simulink model "V3"  (R2024b)
settings: Solver=ode1  StartTime=0.0  StopTime=inf  FixedStep=0.1  RelTol=1e-3  EnableMultiTasking=on
PostLoadFcn:
  | qlabs_setup
model workspace (MAT data in the model file):
  Sig : Simulink.Signal (value not decoded)
  downCamStepSize : Simulink.Parameter (value not decoded)
  lidarStepSize : Simulink.Parameter (value not decoded)
  mainStepSize : Simulink.Parameter (value not decoded)
  mode : Simulink.Parameter (value not decoded)
  realSenseStepSize : Simulink.Parameter (value not decoded)
values from neighbouring files (symbols this model uses):
  map = zeros(mapHeight*pointPerMeter, mapWidth*pointPerMeter)    [map_creator.m]    (also in map_creator_real.m)
  obstacles = [obstacles; coordinateX, coordinateY, rayon;]    [init.m]    (also in init1.m; init_V2.m; init_V3.m; map_creator.m = [)
  pointPerMeter = 50    [map_creator.m]    (also in map_creator_real.m)
  waypoints = [ ... (first row only)    [init.m]    (also in init1.m; init_V2.m; init_V3.m)
  x = input("Veuillez entrer la position x: ")    [map_creator_real.m]
symbols that are objects in the model workspace (value not decoded): downCamStepSize, lidarStepSize, mainStepSize, realSenseStepSize
undefined symbols (not defined in the file or in its folder): DiscIntNeverNeededParam, gcbh, JPEG, Point, qc_get_step_size, Video3D, video_display_show
libraries: quarc_library x30, mpclib x1, simulink_extras x1
(part 2 of 2)

== matlab function V3/LiDAR analysis1/Grid matching ==
  data: map input; x_rob input; y_rob input; scan_ranges input; scan_angles input; theta_opt output double; theta_prec input; pointPerMeter input
function theta_opt = estimate_heading_optimized(map, x_rob, y_rob, scan_ranges, scan_angles, theta_prec, pointPerMeter)
    % map         : Matrice 2D (occupancy grid) avec des valeurs entre 0 et 1
    % x_rob, y_rob: Coordonnées actuelles du robot en mètres 
    % scan_ranges : Vecteur colonne des distances LiDAR (en mètres)
    % scan_angles : Vecteur colonne des angles du LiDAR correspondants (en radians)
    % theta_prec  : Dernier angle connu ou estimé du robot (en radians)
    
    % --- Paramètres fixes ---
    cell_size = 1/pointPerMeter; % 2 cm par case
    [rows, cols] = size(map);
    
    % Centre de la matrice (correspondant à x=0, y=0)
    cx = floor(cols / 2) + 1;
    cy = floor(rows / 2) + 1; 
    
    % --- Espace de recherche restreint ---
    % On cherche de -30° à +30° autour de theta_prec avec un pas de 1°
    % Cela donne exactement 61 valeurs à tester.
    num_steps = 61;
    angle_step = pi / 180; % 1 degré en radians
    start_angle = theta_prec - (30 * angle_step);
    
    max_score = -1;
    theta_opt = theta_prec; % Si le scan est vide, on renvoie l'ancien angle
    
    % --- Boucle de Scan Matching ---
    for i = 1:num_steps
        % Calcul de l'angle testé à la volée (évite les vecteurs de taille variable)
        theta = start_angle + (i - 1) * angle_step;
        current_score = 0;
        
        % On parcourt chaque point du scan LiDAR
        for j = 1:length(scan_ranges)
            range = scan_ranges(j);
            
            % Filtrage des valeurs invalides du capteur (0 ou trop loin)
            if range > 0 && range < 100 
                angle = scan_angles(j);
                
                % 1. Coordonnées globales en mètres
                hit_x_m = x_rob + range * cos(angle + theta);
                hit_y_m = y_rob + range * sin(angle + theta);
                
                % 2. Conversion en indices de la matrice (Y inversé)
                idx_x = cx + round(hit_x_m / cell_size);
                idx_y = cy - round(hit_y_m / cell_size); 
                
                % 3. Vérification des limites pour éviter un crash
                if idx_x >= 1 && idx_x <= cols && idx_y >= 1 && idx_y <= rows
                    % Ajout de la valeur de la case au score de cet angle
                    current_score = current_score + map(idx_y, idx_x);
                end
            end
        end
        
        % 4. Sauvegarde de l'angle si c'est le meilleur score jusqu'à présent
        if current_score > max_score
            max_score = current_score;
            theta_opt = theta;
        end
    end
end

== matlab function V3/LiDAR analysis1/Lidar & Localization/MATLAB Function ==
  data: lidar_position input; ranges input; ranges_c output; angles input; angles_c output
function [ranges_c,angles_c] = correct_lidar(lidar_position, ranges,angles)

x = ranges.*cos(angles) + lidar_position(1);
y = ranges.*sin(angles) + lidar_position(2);

ranges_c = sqrt(x.^2 + y.^2);
angles_c = atan2(y, x);

end

== matlab function V3/MATLAB Function1 ==
  data: t input; X_ref output size=[3, 25]; obstacles input; waypoints input; is_final_approach output
function [X_ref, is_final_approach] = Traj_bezier_horizon(t, obstacles, waypoints)
    % Entrées : 
    %   t          : Temps de simulation actuel (secondes)
    %   obstacles  : Matrice des obstacles [x, y, rayon]
    %   waypoints  : Matrice des points de passage [x, y, theta]
    % Sorties : 
    %   X_ref            : Matrice [3 x Np] contenant les références futures [x; y; theta]
    %   kappa_actuel     : Scalaire de la courbure locale à l'instant t
    %   is_final_approach: Flag (0 ou 1) indiquant l'approche finale

    coder.extrinsic('plot', 'fill', 'quiver', 'figure', 'unwrap', 'warning');

    Ts = 0.1;   % Pas de temps 
    Np = 25;  

    X_ref             = zeros(3, Np);
    kappa_actuel      = 0;
    is_final_approach = 0;

    % Mémoire persistante avec types explicites pour le Coder
    persistent time_ref x_ref y_ref theta_ref kappa_ref initialized

    if isempty(initialized)
        initialized = int32(0);
        v_max = 0.5;
        omega_max = 2.0; 

        obstacles_rect   = [];
        n_points_per_seg = 1000;
        marge_securite   = 0.6;

        % typée double(0x1) pour que le Coder Simulink puisse inférer le type correctement
        x_total     = zeros(0, 1);
        y_total     = zeros(0, 1);
        theta_total = zeros(0, 1);
        kappa_total = zeros(0, 1);
        time_total  = zeros(0, 1);
        cumul_time  = 0;

        for seg = 1:(size(waypoints, 1) - 1)

            x_start = waypoints(seg,   1);  y_start = waypoints(seg,   2);  theta_start = waypoints(seg,   3);
            x_goal  = waypoints(seg+1, 1);  y_goal  = waypoints(seg+1, 2);  theta_goal  = waypoints(seg+1, 3);

            distance = sqrt((x_goal - x_start)^2 + (y_goal - y_start)^2);
            if distance < 1e-3
                warning('Traj_bezier_horizon: segment %d ignoré (distance < 1e-3).', seg);
                continue;
            end

            longueur_tangente = distance / 3;

            P0 = [x_start, y_start];
            P1 = P0 + longueur_tangente * [cos(theta_start), sin(theta_start)];
            P2 = [x_goal, y_goal] - longueur_tangente * [cos(theta_goal), sin(theta_goal)];
            P3 = [x_goal, y_goal];

            % Répulsion des points de contrôle vis-à-vis des obstacles circulaires
            for i = 1:size(obstacles, 1)
                obs_c = obstacles(i, 1:2);
                r_obs = obstacles(i, 3);

                if norm(P1 - obs_c) < r_obs + marge_securite + 0.5
                    dir = (P1 - obs_c) / norm(P1 - obs_c);
                    P1  = obs_c + dir * (r_obs + marge_securite + 0.2);
                end
                if norm(P2 - obs_c) < r_obs + marge_securite + 0.5
                    dir = (P2 - obs_c) / norm(P2 - obs_c);
                    P2  = obs_c + dir * (r_obs + marge_securite + 0.8);
                end
            end

            % Répulsion vis-à-vis des obstacles rectangulaires
            for i = 1:size(obstacles_rect, 1)
                xc  = obstacles_rect(i, 1);  yc  = obstacles_rect(i, 2);
                W   = obstacles_rect(i, 3);  H   = obstacles_rect(i, 4);
                ang = obstacles_rect(i, 5);
                R_mat       = [cos(ang), -sin(ang); sin(ang), cos(ang)];
                corners_loc = [-W/2, -H/2; W/2, -H/2; W/2, H/2; -W/2, H/2];
                corners_glob = (R_mat * corners_loc')' + [xc, yc];
                r_coin = 0.3;

                for j = 1:4
                    coin = corners_glob(j, :);
                    if norm(P1 - coin) < r_coin + marge_securite + 0.5
                        dir = (P1 - coin) / norm(P1 - coin);
                        P1  = coin + dir * (r_coin + marge_securite + 0.8);
                    end
                    if norm(P2 - coin) < r_coin + marge_securite + 0.5
                        dir = (P2 - coin) / norm(P2 - coin);
                        P2  = coin + dir * (r_coin + marge_securite + 0.8);
                    end
                end
            end

            % Génération de la courbe de Bézier cubique
            tt    = linspace(0, 1, n_points_per_seg)';
            x_seg = (1-tt).^3*P0(1) + 3*(1-tt).^2.*tt*P1(1) + 3*(1-tt).*tt.^2*P2(1) + tt.^3*P3(1);
            y_seg = (1-tt).^3*P0(2) + 3*(1-tt).^2.*tt*P1(2) + 3*(1-tt).*tt.^2*P2(2) + tt.^3*P3(2);

            dx  = gradient(x_seg);
            dy  = gradient(y_seg);
            ddx = gradient(dx);
            ddy = gradient(dy);

            theta_seg = atan2(dy, dx);
            kappa     = (dx.*ddy - dy.*ddx) ./ ((dx.^2 + dy.^2).^(3/2) + 1e-6);
            kappa(isnan(kappa)) = 0;

            % Profil de vitesse adaptatif (ralentissement dans les virages)
            v_seg = v_max * ones(size(kappa));
            for k = 1:length(kappa)
                if abs(kappa(k)) > 0.01
                    v_lim    = sqrt(3.0 / abs(kappa(k)));
                    v_seg(k) = min(v_seg(k), v_lim);
                end
            end
            v_seg = min(v_seg, v_max);

            % Conversion paramètre [0,1] → temps réel
            ds       = [0; sqrt(diff(x_seg).^2 + diff(y_seg).^2)];
            dt_seg   = ds ./ max(v_seg, 0.01);
            time_seg = cumsum(dt_seg) + cumul_time;

            if seg == 1
                x_total     = [x_total;     x_seg];     
                y_total     = [y_total;     y_seg];     
                theta_total = [theta_total; theta_seg]; 
                kappa_total = [kappa_total; kappa];     
                time_total  = [time_total;  time_seg]; 
            else
                x_total     = [x_total;     x_seg(2:end)];     
                y_total     = [y_total;     y_seg(2:end)];     
                theta_total = [theta_total; theta_seg(2:end)];
                kappa_total = [kappa_total; kappa(2:end)];     
                time_total  = [time_total;  time_seg(2:end)];  
            end

            cumul_time = time_total(end);
        end
        
        % theta_total = unwrap(theta_total);

        % Stockage persistant
        time_ref  = time_total;
        x_ref     = x_total;
        y_ref     = y_total;
        theta_ref = theta_total;
        kappa_ref = kappa_total;

        % Tracé debug
        figure('Name', 'Trajectoire Bézier MPC', 'Position', [970 100 900 700]);
        hold on; grid on; axis equal;
        for i = 1:size(obstacles, 1)
            circle_x = obstacles(i,1) + obstacles(i,3) * cos(0:0.01:2*pi);
            circle_y = obstacles(i,2) + obstacles(i,3) * sin(0:0.01:2*pi);
            fill(circle_x, circle_y, [1 0.7 0.7], 'EdgeColor', 'r', 'LineWidth', 2);
        end
        plot(x_ref, y_ref, 'b-', 'LineWidth', 3);

        initialized = int32(1);

        % Au tout premier appel on retourne immédiatement les valeurs
        % par défaut déjà initialisées en tête (t=0 → pas encore de
        % trajectoire à interpoler de façon significative).

        return;
    end

    % ==========================================================
    % PHASE 2 : CALCUL DE LA MATRICE DE RÉFÉRENCE SUR L'HORIZON
    % ==========================================================

    % =========================================================
    % ARRÊT : on calcule la distance à l'arrivée en temps réel
    % à partir de la position estimée du robot (x_init passé en
    % entrée depuis le bloc MPC) mais ici on n'a pas x_init.
    % On utilise donc une double condition :
    %   - temporelle  : t > time_ref(end) - marge
    %   - ET spatiale : sera vérifiée côté MPC avec x_init réel
    % On réduit la marge temporelle à 0.5 s (au lieu de 2 s) pour
    % ne déclencher "final" qu'au dernier moment.
    % =========================================================
    dist_to_goal_ref = sqrt((interp1(time_ref, x_ref, min(t, time_ref(end)), 'linear') - x_ref(end))^2 + ...
                            (interp1(time_ref, y_ref, min(t, time_ref(end)), 'linear') - y_ref(end))^2);

    if t > (time_ref(end) - 0.5) || dist_to_goal_ref < 0.3
        is_final_approach = 1;
    else
        is_final_approach = 0;
    end

    if t > time_ref(end)
        % Fin de trajectoire : on reste sur la dernière pose
        X_ref(1, :) = x_ref(end);
        X_ref(2, :) = y_ref(end);
        X_ref(3, :) = theta_ref(end);
        kappa_actuel = 0;
    else
        t_horizon        = t + (0:Np-1) * Ts;
        t_horizon_capped = min(t_horizon, time_ref(end));

        xr_vec     = interp1(time_ref, x_ref,     t_horizon_capped, 'linear');
        yr_vec     = interp1(time_ref, y_ref,     t_horizon_capped, 'linear');
        thetar_vec = interp1(time_ref, theta_ref, t_horizon_capped, 'linear');

        X_ref(1, :) = xr_vec;
        X_ref(2, :) = yr_vec;
        X_ref(3, :) = thetar_vec;

        kappa_actuel = interp1(time_ref, kappa_ref, t, 'spline');
    end
end

== matlab function V3/V1 ==
  data: obstacles input; X_ref input; u_prev input; kappa input; x_init input; u_opt output
function u_opt = Matisse_MPC_Quanser(obstacles, X_ref, u_prev, kappa, x_init)
    % Déclaration pour autoriser les fonctions d'optimisation dans Simulink
    coder.extrinsic('fmincon', 'optimoptions');
    
    % --- Paramètres constants ---
    Np = 12; 
    Ts = 0.1;
    v_max = 0.5;
    w_max = 2.0;
    
    % --- ADAPTATION DYNAMIQUE MATISSE ---
    % 1. Adaptation Géométrique (Courbure)
    Q = diag([10, 10, 5 * (1 + abs(kappa))]); 
    
    % 2. Adaptation Réactive (Obstacles)
    % On cherche la distance à l'obstacle le plus proche
    d_min = 10.0; % Valeur grande par défaut
    if ~isempty(obstacles)
        for j = 1:size(obstacles, 1)
            dist = norm(x_init(1:2) - obstacles(j, 1:2)) - obstacles(j, 3);
            if dist < d_min
                d_min = dist;
            end
        end
    end
    
    % Si l'obstacle est proche, on réduit R pour autoriser une forte accélération
    R_nom = diag([0.1, 0.05]);
    R = R_nom * tanh(max(d_min, 0.1)); 
    
    S = diag([0.5, 0.5]); % Poids sur le lissage (Delta U)
    P = Q * 10;           % Coût terminal pour la stabilité

    % --- BORNES (Limites des moteurs) ---
    % lb et ub doivent être de taille [2*Np, 1]
    lb = repmat([-v_max; -w_max], Np, 1);
    ub = repmat([v_max; w_max], Np, 1);

    % --- OPTIMISATION ---
    % Initialisation avec la commande précédente (Warm Start)
    u0 = repmat(u_prev, Np, 1);
    
    % Options du solveur
    options = optimoptions('fmincon', 'Algorithm', 'sqp', 'Display', 'off');
    
    % Valeur par défaut si fmincon échoue
    u_seq = u0; 
    
    % Appel du solveur (doit être assigné à une variable dans Simulink via coder.extrinsic)
    u_seq = fmincon(@(u) cost_fn(u, x_init, X_ref, u_prev, Q, R, S, P, Np, Ts), ...
                    u0, [], [], [], [], lb, ub, ...
                    @(u) const_fn(u, x_init, obstacles, Np, Ts), options);
                    
    % On ne conserve que la première commande (Horizon Fuyant)
    u_opt = u_seq(1:2);
end

% =========================================================================
% FONCTION DE COÛT (Objectif à minimiser)
% =========================================================================
function J = cost_fn(u_seq, x_init, X_ref, u_prev, Q, R, S, P, Np, Ts)
    J = 0; 
    x = x_init; 
    up = u_prev;
    
    for i = 1:Np
        u = u_seq(2*i-1 : 2*i);
        % Prédiction du modèle cinématique discret
        x = x + [u(1)*cos(x(3)); u(1)*sin(x(3)); u(2)] * Ts;
        
        % Somme : Erreur + Effort + Lissage
        J = J + (x - X_ref(:,i))' * Q * (x - X_ref(:,i)) ...
              + u' * R * u ...
              + (u - up)' * S * (u - up);
        up = u;
    end
    % Ajout du coût terminal
    J = J + (x - X_ref(:,Np))' * P * (x - X_ref(:,Np));
end

% =========================================================================
% FONCTION DE CONTRAINTES NON-LINÉAIRES (LiDAR)
% =========================================================================
function [c, ceq] = const_fn(u_seq, x_init, obstacles, Np, Ts)
    c = [];   % Contraintes d'inégalité (doit être <= 0)
    ceq = []; % Contraintes d'égalité (vide ici)
    
    x = x_init;
    R_robot = 0.2; % Rayon de sécurité autour du QBot
    
    for i = 1:Np
        u = u_seq(2*i-1 : 2*i);
        x = x + [u(1)*cos(x(3)); u(1)*sin(x(3)); u(2)] * Ts;
        
        if ~isempty(obstacles)
            for j = 1:size(obstacles, 1)
                % Distance entre le robot prédit et le centre de l'obstacle
                dist = norm(x(1:2) - obstacles(j, 1:2));
                R_obs = obstacles(j, 3);
                
                % Contrainte : (R_obs + R_robot) - dist <= 0
                % Si la distance est plus petite que la zone de sécurité, c > 0 (violation)
                c = [c; (R_obs + R_robot) - dist]; 
            end
        end
    end
end

== matlab function V3/MATLAB Function3 ==
  data: depth_matrix input; dist_face_obstacle output; bord_gauche output; bord_droite output; alerte_securite output; img_debug output; rgb_matrix input
function [dist_face_obstacle, bord_gauche, bord_droite, alerte_securite, img_debug] = ...
         detecter_obstacles(depth_matrix, rgb_matrix)
% =========================================================================
% Bloc MATLAB Function - Détection d'obstacle par clustering de profondeur
% =========================================================================
% Principe : Dans la ROI centrale, on isole le cluster de pixels dont la
% profondeur est proche du minimum → face avant visible de l'obstacle.
%
% SORTIES :
%   dist_face_obstacle : distance minimale caméra → face avant obstacle (m)
%   bord_gauche        : colonne (px) du bord gauche dans l'image globale
%   bord_droite        : colonne (px) du bord droit dans l'image globale
%   alerte_securite    : true si obstacle détecté sous d_min_alerte (m)
%   img_debug          : matrice depth annotée (cadre ROI + bords obstacle)
%
% ROI centrale : lignes [40%–60%], colonnes [5%–95%] de l'image

    % =====================================================================
    % 1. PARAMÈTRES
    % =====================================================================
    Z_min             = cast(0.15,  'like', depth_matrix); % dist. min valide (m)
    Z_max             = cast(4.0,   'like', depth_matrix); % dist. max valide (m)
    d_min_alerte      = cast(0.4,   'like', depth_matrix); % seuil alerte sécurité (m)
    cluster_tolerance = cast(0.12,  'like', depth_matrix); % tolérance clustering face (m)
    min_cluster_ratio = 0.008; % fraction minimale de pixels ROI pour valider le cluster

    % =====================================================================
    % 2. INITIALISATIONS
    % =====================================================================
    [hauteur, largeur] = size(depth_matrix);

    dist_face_obstacle = Z_max;
    bord_gauche        = cast(0, 'like', depth_matrix);
    bord_droite        = cast(0, 'like', depth_matrix);
    alerte_securite    = false;
    img_debug          = depth_matrix;

    if hauteur < 10 || largeur < 10
        return;
    end

    % =====================================================================
    % 3. NETTOYAGE DE LA MATRICE DE PROFONDEUR
    % =====================================================================
    depth_clean = depth_matrix;
    masque_invalide = isnan(depth_clean)  | ...
                      isinf(depth_clean)  | ...
                      (depth_clean <= 0)  | ...
                      (depth_clean < Z_min) | ...
                      (depth_clean > Z_max);
    depth_clean(masque_invalide) = Z_max;

    % =====================================================================
    % 3.5. FILTRAGE PAR COULEUR (EXEMPLE : DÉTECTION DU ROUGE)
    % =====================================================================
    % Séparation des canaux RGB (l'image est en uint8, de 0 à 255)
    R = rgb_matrix(:,:,1);
    G = rgb_matrix(:,:,2);
    B = rgb_matrix(:,:,3);
    
    % Création d'un masque binaire : 1 si la couleur correspond, 0 sinon
    % faudra ajuster ces seuils selon l'éclairage de la salle en IRL
    seuil_rouge = 150;
    seuil_vert  = 100;
    seuil_bleu  = 100;
    masque_couleur = (R > seuil_rouge) & (G < seuil_vert) & (B < seuil_bleu);
    
    % On force la profondeur à Z_max pour tout ce qui N'EST PAS de la bonne couleur
    depth_clean(~masque_couleur) = Z_max;

    % =====================================================================
    % 4. ROI CENTRALE
    %    rC = [round(hauteur*0.4), round(hauteur*0.6)]
    %    cC = [round(largeur*0.05), round(largeur*0.95)]
    % =====================================================================
    r_start = max(1,       round(hauteur * 0.40));
    r_end   = min(hauteur, round(hauteur * 0.60));
    c_start = max(1,       round(largeur * 0.05));
    c_end   = min(largeur, round(largeur * 0.95));

    roi_C = depth_clean(r_start:r_end, c_start:c_end);
    [roi_h, roi_w] = size(roi_C);

    % =====================================================================
    % 5. CLUSTERING DE LA FACE AVANT DE L'OBSTACLE
    %
    % Inspiré du code MATLAB de clustering fourni :
    % On cherche le pixel le plus proche, puis on regroupe tous les pixels
    % dont la profondeur est dans [d_min, d_min + cluster_tolerance].
    % Ces pixels correspondent à la face plane de l'obstacle en face du robot.
    % =====================================================================

    % --- 5a. Masquer les pixels saturés à Z_max (pas d'obstacle)
    roi_valide = roi_C;
    roi_valide(roi_C >= Z_max) = NaN;

    % --- 5b. Distance minimale dans la ROI (obstacle le plus proche)
    d_min_roi = min(roi_valide(:));

    if isnan(d_min_roi) || isinf(d_min_roi)
        % Aucun obstacle valide dans la ROI → on quitte proprement
        img_debug = dessiner_cadre(img_debug, r_start, r_end, c_start, c_end);
        return;
    end

    % --- 5c. Masque de cluster : pixels appartenant à la face avant
    masque_cluster = (roi_C >= d_min_roi) & ...
                     (roi_C <= (d_min_roi + cluster_tolerance)) & ...
                     (roi_C  < Z_max);

    nb_pixels_cluster = sum(masque_cluster(:));
    nb_pixels_roi     = roi_h * roi_w;

    % Vérification : cluster assez grand pour être un obstacle réel
    if nb_pixels_cluster < round(min_cluster_ratio * nb_pixels_roi)
        img_debug = dessiner_cadre(img_debug, r_start, r_end, c_start, c_end);
        return;
    end

    % =====================================================================
    % 6. DISTANCE LA PLUS PROCHE (point de la face le plus près de la caméra)
    %
    % On prend le MINIMUM (et non la moyenne) pour avoir la distance réelle
    % entre la caméra et le point de surface le plus proche.
    % =====================================================================
    profondeurs_cluster = roi_C(masque_cluster);
    dist_face_obstacle  = cast(min(profondeurs_cluster), 'like', depth_matrix);

    % =====================================================================
    % 7. BORDS GAUCHE ET DROIT DE L'OBSTACLE
    %
    % On projette le masque sur l'axe horizontal.
    % Les colonnes occupées donnent l'emprise latérale de l'obstacle.
    % Conversion locale (dans la ROI) → globale (dans l'image entière).
    % =====================================================================
    cols_occupees = any(masque_cluster, 1); % vecteur 1×roi_w
    indices_cols  = find(cols_occupees);

    if ~isempty(indices_cols)
        bord_gauche = cast(c_start + indices_cols(1)   - 1, 'like', depth_matrix);
        bord_droite = cast(c_start + indices_cols(end) - 1, 'like', depth_matrix);
    end

    % =====================================================================
    % 8. ALERTE SÉCURITÉ — ROI CENTRALE UNIQUEMENT, seuil bas
    % =====================================================================
    if dist_face_obstacle <= d_min_alerte
        alerte_securite = true;
    end

    % =====================================================================
    % 9. TEMPS AVANT COLLISION (TTC) — COMMENTÉ
    %
    % Pour activer, passer la vitesse du robot en paramètre d'entrée.
    %
    % v_robot = 0.5;  % vitesse de déplacement du robot (m/s)
    % if v_robot > 0 && dist_face_obstacle < Z_max
    %     TTC = dist_face_obstacle / v_robot;
    %     % TTC en secondes. Si TTC < seuil_urgence → évitement immédiat.
    %     % Exemple : seuil_urgence = 1.5 s
    % else
    %     TTC = inf;
    % end
    %
    % NOTE : Pour plus de précision, utiliser la dérivée temporelle
    % de dist_face_obstacle entre deux frames :
    %   v_approche = (dist_prev - dist_face_obstacle) / dt;
    %   TTC = dist_face_obstacle / v_approche;  (si v_approche > 0)
    % =====================================================================

    % =====================================================================
    % 10. ESTIMATION ANGULAIRE DES BORDS (nécessite calibration caméra)
    %
    % Si tu connais la focale horizontale fx et le centre optique cx :
    %
    % fx = 462.0;  % pixels (valeur typique pour caméra QBot)
    % cx = largeur / 2;
    %
    % angle_bord_gauche = atan2d(double(bord_gauche) - cx, fx);  % degrés
    % angle_bord_droite = atan2d(double(bord_droite) - cx, fx);
    %
    % dist_laterale_gauche = dist_face_obstacle * tand(angle_bord_gauche);
    % dist_laterale_droite = dist_face_obstacle * tand(angle_bord_droite);
    % Ces distances en mètres indiquent l'offset latéral des bords.
    % =====================================================================

    % =====================================================================
    % 11. IMAGE DE DÉBOGAGE
    % =====================================================================
    % Cadre noir de la ROI
img_debug = dessiner_cadre(img_debug, r_start, r_end, c_start, c_end);

% --- BORDS DE L'OBSTACLE EN BLANC ---
% Valeur 10.0 = pixel blanc/brillant après normalisation (/10) pour le Video Viewer
    if bord_gauche > 0 && bord_droite > 0
        col_g = min(largeur, max(1, round(double(bord_gauche))));
        col_d = min(largeur, max(1, round(double(bord_droite))));
    
        % Ligne verticale blanche sur toute la hauteur de la ROI
        for r = r_start:r_end
            img_debug(r, col_g) = cast(10.0, 'like', depth_matrix); % bord gauche blanc
            img_debug(r, col_d) = cast(10.0, 'like', depth_matrix); % bord droit blanc
        end
    end

end % fin fonction principale

% =========================================================================
% SOUS-FONCTION : Dessin du cadre de la ROI
% =========================================================================
function img = dessiner_cadre(img, r_start, r_end, c_start, c_end)
    img(r_start:r_end, c_start) = 0;  % bord gauche ROI (noir)
    img(r_start:r_end, c_end)   = 0;  % bord droit ROI
    img(r_start, c_start:c_end) = 0;  % bord haut ROI
    img(r_end,   c_start:c_end) = 0;  % bord bas ROI
end

== matlab function V3/V2 ==
  data: x_init input size=[3,1]; X_ref input size=[3, 25]; u_prev input size=[2, 1]; obstacles input; kappa input; u_opt output; is_final input
% function u_opt = Matisse_MPC_Quanser(x_init, X_ref, u_prev, obstacles, kappa)
% function u_opt = Matisse_MPC_Quanser(x_init, X_ref, u_prev, obstacles, kappa)
%     % On déclare uniquement notre nouveau fichier comme extrinsic
%     coder.extrinsic('solve_mpc_matisse');
% 
%     % --- Paramètres ---
%     Np = 25; 
%     Ts = 0.1;
%     v_max = 0.5;
%     w_max = 2.0;
% 
%     % --- SOLUTION À L'ERREUR "Underspecified Dimensions" ---
%     % On pré-alloue les variables pour que le compilateur C connaisse leurs tailles
%     u_seq = zeros(2*Np, 1);
%     u_opt = zeros(2, 1);
% 
%     % --- ADAPTATION DYNAMIQUE ---
%     % Q = diag([10, 10, 5 * (1 + abs(kappa))]); 
%     Q = diag([1, 1, 0.5]);
%     d_min = 10.0;
%     if ~isempty(obstacles)
%         for j = 1:size(obstacles, 1)
%             dist = norm(x_init(1:2) - obstacles(j, 1:2)) - obstacles(j, 3);
%             if dist < d_min
%                 d_min = dist;
%             end
%         end
%     end
% 
%     % R_nom = diag([0.1, 0.05]);
%     % R = R_nom * tanh(max(d_min, 0.1)); 
%     R = diag([0.05, 0.05]);
%     S = diag([0.5, 2.0]); 
%     P = Q;           
% 
%     lb = repmat([-v_max; -w_max], Np, 1);
%     ub = repmat([v_max; w_max], Np, 1);
%     u0 = repmat(u_prev, Np, 1);
% 
%     % --- APPEL À L'OPTIMISEUR EXTERNE ---
%     % Plus de fonction avec @(u) ici, tout est géré par MATLAB dans le fichier .m
%     u_seq = solve_mpc_matisse(x_init, X_ref, u_prev, Q, R, S, P, Np, Ts, obstacles, lb, ub, u0);
% 
%     % Extraction de la commande
%     u_opt = u_seq(1:2);
% end



% function u_opt = Matisse_MPC_Quanser(x_init, X_ref, u_prev, obstacles, kappa)
% 
%     coder.extrinsic('solve_mpc_matisse');
% 
%     % --- Paramètres (Synchronisés) ---
%     Np = 25; 
%     Ts = 0.1;
%     v_max = 0.5;
%     w_max = 2.0;
% 
%     % --- Pré-allocation ---
%     u_seq = zeros(2*Np, 1);
%     u_opt = zeros(2, 1);
% 
%     % --- Matrices de Pondération ---
%     Q = diag([10, 10, 0.1]);   % Suivi de trajectoire souple
%     R = diag([0.1, 0.1]);  % Coût de l'effort
%     S = diag([1, 5]);    % Lissage (Anti-zigzag)
%     P = Q;                   % Coût terminal
% 
%     % --- Bornes et Initialisation ---
%     lb = repmat([-v_max; -w_max], Np, 1);
%     ub = repmat([v_max; w_max], Np, 1);
%     u0 = repmat([0.1; 0], Np, 1); % On lui suggère d'avancer un tout petit peu
% 
% 
% 
% 
%     % --- Appel à l'Optimiseur Externe ---
%     u_seq = solve_mpc_matisse(x_init, X_ref, u_prev, Q, R, S, P, Np, Ts, obstacles, lb, ub, u0);
% 
%     u_opt = u_seq(1:2);
% end

function u_opt = Matisse_MPC_Quanser(x_init, X_ref, u_prev, obstacles, kappa, is_final)
    % IMPORTANT : "is_final" doit être écrit ci-dessus dans la liste des arguments !
    
    coder.extrinsic('solve_mpc_matisse');
    
    % --- Paramètres ---
    Np = 25; 
    Ts = 0.1;
    v_max = 0.5;
    w_max = 2.0;
    
    % --- Pré-allocation ---
    u_seq = zeros(2*Np, 1);
    u_opt = zeros(2, 1);
    
    % --- Matrices de Pondération ---
    Q = diag([10, 10, 0.1]);   
    R = diag([0.1, 0.1]);
    S = diag([1, 5]);
    
    % --- CALCUL DE LA DISTANCE (On la définit ICI avant le IF) ---
    dist_final = norm(x_init(1:2) - X_ref(1:2, end));

    % --- LOGIQUE D'ARRÊT ---
    if is_final == 1 && dist_final < 0.1
        u_opt = [0; 0]; % On force l'arrêt
    else
        % On ajuste Q si on est en approche finale pour éviter de "vriller"
        if is_final == 1
            Q(3,3) = 0.01; 
        end
        
        P = Q;
        lb = repmat([-v_max; -w_max], Np, 1);
        ub = repmat([v_max; w_max], Np, 1);
        u0 = repmat([0.1; 0], Np, 1); 
        
        % Appel à l'optimiseur
        u_seq = solve_mpc_matisse(x_init, X_ref, u_prev, Q, R, S, P, Np, Ts, obstacles, lb, ub, u0);
        u_opt = u_seq(1:2);
    end
end

== matlab function V3/MATLAB Function2 ==
  data: t input; X_ref output size=[3, 25]; kappa_actuel output; obstacles input size=[1, 3]; waypoints input size=[5, 3]; is_final_approach output
function [X_ref, kappa_actuel, is_final_approach] = Traj_bezier_horizon(t, obstacles, waypoints)
    % Entrées : 
    %   t : Temps de simulation actuel (secondes)
    %   obstacles : Matrice des obstacles [x, y, rayon]
    %   waypoints : Matrice des points de passage [x, y, theta]
    % Sorties : 
    %   X_ref : Matrice [3 x Np] contenant les références futures [x; y; theta]
    %   kappa_actuel : Scalaire de la courbure locale à l'instant t

    coder.extrinsic('plot', 'fill', 'quiver', 'figure');
    
    % --- Paramètres MPC (À ajuster selon le solveur utilisé) ---
    Ts = 0.1;   % Pas de temps d'échantillonnage (100 ms)
    Np = 25;    % Horizon de prédiction (1.2 secondes dans le futur)
    
    % Mémoire persistante pour ne calculer la trajectoire qu'une seule fois
    persistent time_ref x_ref y_ref theta_ref kappa_ref initialized
    
    if isempty(initialized)
        v_max = 0.3;           
        omega_max = 2.0;       
        
        % Obstacles Rectangulaires [x, y, w, h, theta]
        obstacles_rect = [];
        
        n_points_per_seg = 1000; % Points par segment
        marge_securite = 0.6;

        % Initialisation des vecteurs totaux
        x_total = []; y_total = []; theta_total = [];
        kappa_total = []; time_total = []; % <--- AJOUT KAPPA
        
        cumul_time = 0;
        
        % Boucle sur chaque segment (entre waypoint i et i+1)
        for seg = 1:(size(waypoints, 1) - 1)
            
            x_start = waypoints(seg, 1); y_start = waypoints(seg, 2); theta_start = waypoints(seg, 3);
            x_goal = waypoints(seg+1, 1); y_goal = waypoints(seg+1, 2); theta_goal = waypoints(seg+1, 3);
            
            % Tangentes -> points intermédiaires
            distance = sqrt((x_goal - x_start)^2 + (y_goal - y_start)^2);
            longueur_tangente = distance / 3;
             
            P0 = [x_start, y_start];
            P1 = P0 + longueur_tangente * [cos(theta_start), sin(theta_start)];
            P2 = [x_goal, y_goal] - longueur_tangente * [cos(theta_goal), sin(theta_goal)];
            P3 = [x_goal, y_goal];
            
            % On modifie les points intermédiaires s'ils sont trop proche d'un obstacle
            for i = 1:size(obstacles, 1)
                obs_c = obstacles(i, 1:2); r_obs = obstacles(i, 3);
                
                % P1
                if norm(P1 - obs_c) < r_obs + marge_securite + 0.5
                    dir = (P1 - obs_c) / norm(P1 - obs_c);
                    P1 = obs_c + dir * (r_obs + marge_securite + 0.2);
                end
                % P2
                if norm(P2 - obs_c) < r_obs + marge_securite + 0.5
                    dir = (P2 - obs_c) / norm(P2 - obs_c);
                    P2 = obs_c + dir * (r_obs + marge_securite + 0.8);
                end
            end
            
            for i = 1:size(obstacles_rect, 1)
                xc = obstacles_rect(i, 1); yc = obstacles_rect(i, 2);
                W = obstacles_rect(i, 3); H = obstacles_rect(i, 4); ang = obstacles_rect(i, 5);
                R_mat = [cos(ang), -sin(ang); sin(ang), cos(ang)];
                corners_loc = [-W/2, -H/2; W/2, -H/2; W/2, H/2; -W/2, H/2];
                corners_glob = (R_mat * corners_loc')' + [xc, yc];
                r_coin = 0.3;
                
                % Vérifier P1 et P2 contre les 4 coins
                for j=1:4
                    coin = corners_glob(j,:);
                    if norm(P1 - coin) < r_coin + marge_securite + 0.5
                         dir = (P1 - coin)/norm(P1 - coin);
                         P1 = coin + dir * (r_coin + marge_securite + 0.8);
                    end
                    if norm(P2 - coin) < r_coin + marge_securite + 0.5
                         dir = (P2 - coin)/norm(P2 - coin);
                         P2 = coin + dir * (r_coin + marge_securite + 0.8);
                    end
                end
            end
            
            % génération de la trajectoire via Bezier
            tt = linspace(0, 1, n_points_per_seg)';
            x_seg = (1-tt).^3*P0(1) + 3*(1-tt).^2.*tt*P1(1) + 3*(1-tt).*tt.^2*P2(1) + tt.^3*P3(1);
            y_seg = (1-tt).^3*P0(2) + 3*(1-tt).^2.*tt*P1(2) + 3*(1-tt).*tt.^2*P2(2) + tt.^3*P3(2);
            
            dx = gradient(x_seg); dy = gradient(y_seg);
            theta_seg = atan2(dy, dx);
            
            ddx = gradient(dx); ddy = gradient(dy);
            kappa = (dx.*ddy - dy.*ddx) ./ ((dx.^2 + dy.^2).^(3/2) + 1e-6);
            kappa(isnan(kappa)) = 0;
            
            % Profil de vitesse
            v_seg = v_max * ones(size(kappa));
            for k=1:length(kappa)
                if abs(kappa(k)) > 0.01 % si la courbure est trop elevee on ralentit
                    v_lim = sqrt(3.0 / abs(kappa(k)));
                    v_seg(k) = min(v_seg(k), v_lim);
                end
            end
            v_seg = min(v_seg, v_max);
            
            % conversion du temps de bezier ([0,1]) en un temps reel base sur v_seg
            ds = sqrt(diff(x_seg).^2 + diff(y_seg).^2);
            ds = [0; ds];
            dt = ds ./ max(v_seg, 0.01);
            time_seg = cumsum(dt) + cumul_time;

            if seg == 1
                x_total = [x_total; x_seg];
                y_total = [y_total; y_seg];
                theta_total = [theta_total; theta_seg];
                kappa_total = [kappa_total; kappa]; % <--- AJOUT IMPORTANT
                time_total = [time_total; time_seg];
            else
                % On saute le premier point pour éviter les doublons
                x_total = [x_total; x_seg(2:end)];
                y_total = [y_total; y_seg(2:end)];
                theta_total = [theta_total; theta_seg(2:end)];
                kappa_total = [kappa_total; kappa(2:end)]; % <--- AJOUT IMPORTANT
                time_total = [time_total; time_seg(2:end)];
            end
            
            cumul_time = time_total(end);
        end
        
        % Correction finale des angles (Unwrap) pour éviter les sauts +/- Pi
        theta_total = unwrap(theta_total);

        % Stockage Persistant
        time_ref = time_total;
        x_ref = x_total;
        y_ref = y_total;
        theta_ref = theta_total;
        kappa_ref = kappa_total; % <--- AJOUT IMPORTANT

        % --- GESTION DU TRACÉ (Facultatif mais utile pour le debug) ---
        figure('Name', 'Trajectoire Bézier MPC', 'Position', [970 100 900 700]);
        hold on; grid on; axis equal;
        for i = 1:size(obstacles, 1)
            circle_x = obstacles(i,1) + obstacles(i,3) * cos(0:0.01:2*pi);
            circle_y = obstacles(i,2) + obstacles(i,3) * sin(0:0.01:2*pi);
            fill(circle_x, circle_y, [1 0.7 0.7], 'EdgeColor', 'r', 'LineWidth', 2);
        end
        plot(x_ref, y_ref, 'b-', 'LineWidth', 3);
        % ... (Tu peux garder ton code de dessin des waypoints ici si tu veux)
        
        initialized = 1;
    end
    
    % ==========================================================
    % PHASE 2 : CALCUL DE LA MATRICE DE RÉFÉRENCE SUR L'HORIZON
    % ==========================================================
    
%     % Initialisation de la matrice de sortie (obligatoire pour le coder Simulink)
%     X_ref = zeros(3, Np);
% 
%     if t > time_ref(end)
%         % Fin de la trajectoire : on reste sur place
%         X_ref(1, :) = x_ref(end);
%         X_ref(2, :) = y_ref(end);
%         X_ref(3, :) = theta_ref(end);
%         kappa_actuel = 0;
%     else
%         % 1. Création du vecteur de temps futur [t, t+Ts, t+2Ts, ..., t+(Np-1)Ts]
%         t_horizon = t + (0 : Np-1) * Ts;
% 
%         % 2. Plafonnement du temps pour ne pas déborder du tableau
%         t_horizon_capped = min(t_horizon, time_ref(end));
% 
%         % 3. Interpolation Vectorielle
%         % On interpole la position désirée pour tous les points de l'horizon
%         xr_vec = interp1(time_ref, x_ref, t_horizon_capped, 'linear');
%         yr_vec = interp1(time_ref, y_ref, t_horizon_capped, 'linear');
%         thetar_vec = interp1(time_ref, theta_ref, t_horizon_capped, 'linear');
% 
%         % 4. Remplissage de la matrice de sortie
%         X_ref(1, :) = xr_vec;
%         X_ref(2, :) = yr_vec;
%         X_ref(3, :) = thetar_vec;
% 
%         % 5. Extraction de la courbure à l'instant présent t
%         kappa_actuel = interp1(time_ref, kappa_ref, t, 'spline');
%     end
% end

    % --- À modifier dans la PHASE 2 ---
    X_ref = zeros(3, 25); % Np = 25
    Ts = 0.1;
    Np = 25;
    
    % On détecte si on est dans les dernières secondes du trajet
    if t > (time_ref(end) - 2.0) % On active la vigilance 2 secondes avant la fin théorique
        is_final_approach = 1;
    else
        is_final_approach = 0;
    end

    if t > time_ref(end)
        X_ref(1, :) = x_ref(end);
        X_ref(2, :) = y_ref(end);
        X_ref(3, :) = theta_ref(end);
        kappa_actuel = 0;
    else
        t_horizon = t + (0 : Np-1) * Ts;
        t_horizon_capped = min(t_horizon, time_ref(end));
        
        xr_vec = interp1(time_ref, x_ref, t_horizon_capped, 'linear');
        yr_vec = interp1(time_ref, y_ref, t_horizon_capped, 'linear');
        thetar_vec = interp1(time_ref, theta_ref, t_horizon_capped, 'linear');
        
        X_ref(1, :) = xr_vec;
        X_ref(2, :) = yr_vec;
        X_ref(3, :) = thetar_vec;
        
        kappa_actuel = interp1(time_ref, kappa_ref, t, 'spline');
    end
end

== matlab function V3/nouv LiDAR analysis2/Grid matching ==
  data: map input; x_rob input; y_rob input; ranges input; angles input; theta output double; pointPerMeter input; previousTheta input
function theta = estimate_theta(map, x_rob, y_rob, ranges, angles, pointPerMeter, previousTheta)
    %#codegen
    % Note : x_rob et y_rob représentent ici la position du LiDAR, 
    % l'offset ayant été géré en amont dans le schéma Simulink.
    
    % --- Paramètres ---
    [mapRows, mapCols] = size(map);
    % On suppose que le centre de la matrice correspond aux coordonnées (0,0)
    center_row = mapRows / 2;
    center_col = mapCols / 2;
    
    % --- Filtrage des mesures LiDAR ---
    valid_idx = (ranges > 0) & (ranges < inf);
    r_valid = ranges(valid_idx);
    a_valid = angles(valid_idx);
    
    % --- Recherche de l'angle optimal (Scan Matching) ---
    % Test des angles de -pi à pi avec une résolution de 1 degré
    theta_search = -pi : (pi/180) : pi; 
    
    best_score = -1;
    best_theta = 0;
    
    % Boucle sur chaque angle possible
    for i = 1:length(theta_search)
        t = theta_search(i);
        
        % 1. Projection des points LiDAR dans le repère global
        % L'angle global du rayon est l'angle local du LiDAR + l'angle testé (t)
        x_pts = x_rob + r_valid .* cos(a_valid + t);
        y_pts = y_rob + r_valid .* sin(a_valid + t);
        
        % 2. Conversion des coordonnées monde (m) en indices de matrice (pixels)
        cols = round(center_col + (x_pts * pointPerMeter));
        rows = round(center_row - (y_pts * pointPerMeter)); 
        
        % 3. Filtrage de sécurité : on ignore les points hors de la carte
        in_bounds = (rows >= 1) & (rows <= mapRows) & (cols >= 1) & (cols <= mapCols);
        rows_in = rows(in_bounds);
        cols_in = cols(in_bounds);
        
        % 4. Calcul du score
        if isempty(rows_in)
            score = 0;
        else
            % Score = somme des "probabilités" d'obstacle sur la carte
            linear_indices = sub2ind([mapRows, mapCols], rows_in, cols_in);
            score = sum(map(linear_indices));
        end
        
        % 5. Mémorisation du meilleur angle
        if score > best_score
            best_score = score;
            best_theta = t;
        end
    end
    
    % Sortie finale (seulement si le theta est cohérent)
    difference = rad2deg(previousTheta-best_theta);
    if difference >= -45 && difference <= 45
        theta = best_theta;
    else
        theta = previousTheta;
    end
end

== matlab function V3/Extended Kalman filter/MATLAB Function ==
  data: v input; X_pred output; w input; xk input; yk input; thetak input; P input; Y_pred output; theta_pred output; P_pred output
function [X_pred, Y_pred, theta_pred, P_pred] = prediction(v, w, xk, yk, thetak, P)
    Ts = 0.01;
    
    % Vecteur d'état actuel
    X = [xk; yk; thetak];
   
    % 1. MODÈLE D'ÉTAT (Cinématique du QBot)
    % On calcule la prédiction basée sur les vitesses v (linéaire) et w (angulaire)
    X_next = X + [v * cos(thetak) * Ts;
                  v * sin(thetak) * Ts;
                  w * Ts];
    
    % Extraction des sorties
    X_pred     = X_next(1);
    Y_pred     = X_next(2);
    % theta_pred = atan2(sin(X_next(3)), cos(X_next(3))); % Normalisation d'angle (-pi à pi)
    theta_pred = atan2(sin(X_next(3)), cos(X_next(3))); %CHANGEMENT
    %theta_pred =X_next(3);

    % 2. LINÉARISATION (Calcul de la Jacobienne F)
    % f est la dérivée de l'équation d'état par rapport à x, y et theta
    F = [1, 0, -v * Ts * sin(thetak);
         0, 1,  v * Ts *cos(thetak);
         0, 0,  1];

    % 3. BRUIT DE MODÈLE (Matrice Q)
    % Plus ces valeurs sont élevées, moins on fait confiance au modèle théorique
    % À ajuster
    q_x = 0.001; %0.00001; %0.001
    q_y = 0.001; %0.00001;%0.001
    q_theta = 0.001; %0.00002;%0.002
    Q = diag([q_x, q_y, q_theta]);

    % 4. PRÉDICTION DE LA COVARIANCE
    % On propage l'incertitude P_pred = F*P*F' + Q
    P_pred = F * P * F' + Q;
end
